simulink library "xrbsMath_r3"  (Simulink 5.0)
undefined symbols (not defined in the file or in its folder): num_width
libraries: xbsIndex_r3 x775, xrbsMath_r3 x16
(part 7 of 8)

== system xrbsMath_r3/CORDIC DIVIDER/Quadrant Map/Normalize X/Shift15 ==
  din : Inport
  cin : Inport  Port=2
  msb : Inport  Port=3
  AddSub : xbsIndex_r3/AddSub  mode=Addition  precision=Full  arith_type=Unsigned  n_bits=8  bin_pt=2  quantization=Truncate  overflow=Wrap  latency=1  explicit_period=off  period=1  en=off  dbl_ovrd=off  use_core=on  pipeline=off  use_rpm=off  gen_core=on
      settings: xl_area=[2 3 0 2 0 0 0]
  Inverter : xbsIndex_r3/Inverter  latency=0  explicit_period=off  period=1  en=off  dbl_ovrd=off
      settings: xl_area=[1 0 0 1 0 0 0]
  Inverter1 : xbsIndex_r3/Inverter  latency=0  explicit_period=off  period=1  en=off  dbl_ovrd=off
      settings: xl_area=[1 0 0 1 0 0 0]
  Logical : xbsIndex_r3/Logical  logical_function=AND  inputs=2  precision=Full  arith_type=Unsigned  n_bits=8  bin_pt=2  align_bp=on  latency=0  explicit_period=off  period=1  en=off  dbl_ovrd=off
      settings: xl_area=[1 0 0 1 0 0 0]
  Logical1 : xbsIndex_r3/Logical  logical_function=OR  inputs=2  precision=Full  arith_type=Unsigned  n_bits=8  bin_pt=2  align_bp=on  latency=0  explicit_period=off  period=1  en=off  dbl_ovrd=off
      settings: xl_area=[1 0 0 1 0 0 0]
  Mux : xbsIndex_r3/Mux  inputs=2  precision=Full  arith_type="Signed  (2's comp)"  n_bits=8  bin_pt=2  quantization=Truncate  overflow=Wrap  latency=1  mux_type=off  explicit_period=off  period=1  en=off  dbl_ovrd=off  use_rpm=off  gen_core=on
      settings: xl_area=[8 15 0 15 0 0 0]
  Register : xbsIndex_r3/Register  init=0  reg_only_valid=off  explicit_period=off  period=1  rst=off  en=off  out_en=off  dbl_ovrd=off
      settings: xl_area=[1 1 0 0 0 0 0]
  Shift : xbsIndex_r3/Shift  shift_dir=Left  shift_bits=1  precision=User Defined  arith_type=Unsigned  n_bits=num_bits  bin_pt=bin_point  quantization=Truncate  overflow=Wrap  latency=0  explicit_period=off  period=1  en=off  dbl_ovrd=off
      settings: xl_area=[0 0 0 0 0 0 0]
  Slice : xbsIndex_r3/Slice  mode=Upper Bit Location + Width  nbits=1  bit1=0  base1=MSB of Input  bit0=0  base0=LSB of Input  boolean_output=off  explicit_period=off  period=1  dbl_ovrd=off
  dout : Outport
  sum : Outport  Port=2
  latch : Outport  Port=3
  wires:
  Register/1 -> latch/1
  Shift/1 -> Mux/2
  Mux/1 -> dout/1
  Logical1/1 -> Mux/1, Register/1
  Logical/1 -> AddSub/1
  Inverter1/1 -> Logical/2
  msb/1 -> Logical1/2, Inverter1/1
  Inverter/1 -> Logical/1
  cin/1 -> AddSub/2
  AddSub/1 -> sum/1
  din/1 -> Mux/3, Shift/1, Slice/1
  Slice/1 -> Logical1/1, Inverter/1

== system xrbsMath_r3/CORDIC DIVIDER/Quadrant Map/Normalize X/Shift2 ==
  din : Inport
  cin : Inport  Port=2
  msb : Inport  Port=3
  AddSub : xbsIndex_r3/AddSub  mode=Addition  precision=Full  arith_type=Unsigned  n_bits=8  bin_pt=2  quantization=Truncate  overflow=Wrap  latency=1  explicit_period=off  period=1  en=off  dbl_ovrd=off  use_core=on  pipeline=off  use_rpm=off  gen_core=on
      settings: xl_area=[2 3 0 2 0 0 0]
  Inverter : xbsIndex_r3/Inverter  latency=0  explicit_period=off  period=1  en=off  dbl_ovrd=off
      settings: xl_area=[1 0 0 1 0 0 0]
  Inverter1 : xbsIndex_r3/Inverter  latency=0  explicit_period=off  period=1  en=off  dbl_ovrd=off
      settings: xl_area=[1 0 0 1 0 0 0]
  Logical : xbsIndex_r3/Logical  logical_function=AND  inputs=2  precision=Full  arith_type=Unsigned  n_bits=8  bin_pt=2  align_bp=on  latency=0  explicit_period=off  period=1  en=off  dbl_ovrd=off
      settings: xl_area=[1 0 0 1 0 0 0]
  Logical1 : xbsIndex_r3/Logical  logical_function=OR  inputs=2  precision=Full  arith_type=Unsigned  n_bits=8  bin_pt=2  align_bp=on  latency=0  explicit_period=off  period=1  en=off  dbl_ovrd=off
      settings: xl_area=[1 0 0 1 0 0 0]
  Mux : xbsIndex_r3/Mux  inputs=2  precision=Full  arith_type="Signed  (2's comp)"  n_bits=8  bin_pt=2  quantization=Truncate  overflow=Wrap  latency=1  mux_type=off  explicit_period=off  period=1  en=off  dbl_ovrd=off  use_rpm=off  gen_core=on
      settings: xl_area=[8 15 0 15 0 0 0]
  Register : xbsIndex_r3/Register  init=0  reg_only_valid=off  explicit_period=off  period=1  rst=off  en=off  out_en=off  dbl_ovrd=off
      settings: xl_area=[1 1 0 0 0 0 0]
  Shift : xbsIndex_r3/Shift  shift_dir=Left  shift_bits=1  precision=User Defined  arith_type=Unsigned  n_bits=num_bits  bin_pt=bin_point  quantization=Truncate  overflow=Wrap  latency=0  explicit_period=off  period=1  en=off  dbl_ovrd=off
      settings: xl_area=[0 0 0 0 0 0 0]
  Slice : xbsIndex_r3/Slice  mode=Upper Bit Location + Width  nbits=1  bit1=0  base1=MSB of Input  bit0=0  base0=LSB of Input  boolean_output=off  explicit_period=off  period=1  dbl_ovrd=off
  dout : Outport
  sum : Outport  Port=2
  latch : Outport  Port=3
  wires:
  Register/1 -> latch/1
  Shift/1 -> Mux/2
  Mux/1 -> dout/1
  Logical1/1 -> Mux/1, Register/1
  Logical/1 -> AddSub/1
  Inverter1/1 -> Logical/2
  msb/1 -> Logical1/2, Inverter1/1
  Inverter/1 -> Logical/1
  cin/1 -> AddSub/2
  AddSub/1 -> sum/1
  din/1 -> Mux/3, Shift/1, Slice/1
  Slice/1 -> Logical1/1, Inverter/1

== system xrbsMath_r3/CORDIC DIVIDER/Quadrant Map/Normalize X/Shift3 ==
  din : Inport
  cin : Inport  Port=2
  msb : Inport  Port=3
  AddSub : xbsIndex_r3/AddSub  mode=Addition  precision=Full  arith_type=Unsigned  n_bits=8  bin_pt=2  quantization=Truncate  overflow=Wrap  latency=1  explicit_period=off  period=1  en=off  dbl_ovrd=off  use_core=on  pipeline=off  use_rpm=off  gen_core=on
      settings: xl_area=[2 3 0 2 0 0 0]
  Inverter : xbsIndex_r3/Inverter  latency=0  explicit_period=off  period=1  en=off  dbl_ovrd=off
      settings: xl_area=[1 0 0 1 0 0 0]
  Inverter1 : xbsIndex_r3/Inverter  latency=0  explicit_period=off  period=1  en=off  dbl_ovrd=off
      settings: xl_area=[1 0 0 1 0 0 0]
  Logical : xbsIndex_r3/Logical  logical_function=AND  inputs=2  precision=Full  arith_type=Unsigned  n_bits=8  bin_pt=2  align_bp=on  latency=0  explicit_period=off  period=1  en=off  dbl_ovrd=off
      settings: xl_area=[1 0 0 1 0 0 0]
  Logical1 : xbsIndex_r3/Logical  logical_function=OR  inputs=2  precision=Full  arith_type=Unsigned  n_bits=8  bin_pt=2  align_bp=on  latency=0  explicit_period=off  period=1  en=off  dbl_ovrd=off
      settings: xl_area=[1 0 0 1 0 0 0]
  Mux : xbsIndex_r3/Mux  inputs=2  precision=Full  arith_type="Signed  (2's comp)"  n_bits=8  bin_pt=2  quantization=Truncate  overflow=Wrap  latency=1  mux_type=off  explicit_period=off  period=1  en=off  dbl_ovrd=off  use_rpm=off  gen_core=on
      settings: xl_area=[8 15 0 15 0 0 0]
  Register : xbsIndex_r3/Register  init=0  reg_only_valid=off  explicit_period=off  period=1  rst=off  en=off  out_en=off  dbl_ovrd=off
      settings: xl_area=[1 1 0 0 0 0 0]
  Shift : xbsIndex_r3/Shift  shift_dir=Left  shift_bits=1  precision=User Defined  arith_type=Unsigned  n_bits=num_bits  bin_pt=bin_point  quantization=Truncate  overflow=Wrap  latency=0  explicit_period=off  period=1  en=off  dbl_ovrd=off
      settings: xl_area=[0 0 0 0 0 0 0]
  Slice : xbsIndex_r3/Slice  mode=Upper Bit Location + Width  nbits=1  bit1=0  base1=MSB of Input  bit0=0  base0=LSB of Input  boolean_output=off  explicit_period=off  period=1  dbl_ovrd=off
  dout : Outport
  sum : Outport  Port=2
  latch : Outport  Port=3
  wires:
  Register/1 -> latch/1
  Shift/1 -> Mux/2
  Mux/1 -> dout/1
  Logical1/1 -> Mux/1, Register/1
  Logical/1 -> AddSub/1
  Inverter1/1 -> Logical/2
  msb/1 -> Logical1/2, Inverter1/1
  Inverter/1 -> Logical/1
  cin/1 -> AddSub/2
  AddSub/1 -> sum/1
  din/1 -> Mux/3, Shift/1, Slice/1
  Slice/1 -> Logical1/1, Inverter/1

== system xrbsMath_r3/CORDIC DIVIDER/Quadrant Map/Normalize X/Shift4 ==
  din : Inport
  cin : Inport  Port=2
  msb : Inport  Port=3
  AddSub : xbsIndex_r3/AddSub  mode=Addition  precision=Full  arith_type=Unsigned  n_bits=8  bin_pt=2  quantization=Truncate  overflow=Wrap  latency=1  explicit_period=off  period=1  en=off  dbl_ovrd=off  use_core=on  pipeline=off  use_rpm=off  gen_core=on
      settings: xl_area=[2 3 0 2 0 0 0]
  Inverter : xbsIndex_r3/Inverter  latency=0  explicit_period=off  period=1  en=off  dbl_ovrd=off
      settings: xl_area=[1 0 0 1 0 0 0]
  Inverter1 : xbsIndex_r3/Inverter  latency=0  explicit_period=off  period=1  en=off  dbl_ovrd=off
      settings: xl_area=[1 0 0 1 0 0 0]
  Logical : xbsIndex_r3/Logical  logical_function=AND  inputs=2  precision=Full  arith_type=Unsigned  n_bits=8  bin_pt=2  align_bp=on  latency=0  explicit_period=off  period=1  en=off  dbl_ovrd=off
      settings: xl_area=[1 0 0 1 0 0 0]
  Logical1 : xbsIndex_r3/Logical  logical_function=OR  inputs=2  precision=Full  arith_type=Unsigned  n_bits=8  bin_pt=2  align_bp=on  latency=0  explicit_period=off  period=1  en=off  dbl_ovrd=off
      settings: xl_area=[1 0 0 1 0 0 0]
  Mux : xbsIndex_r3/Mux  inputs=2  precision=Full  arith_type="Signed  (2's comp)"  n_bits=8  bin_pt=2  quantization=Truncate  overflow=Wrap  latency=1  mux_type=off  explicit_period=off  period=1  en=off  dbl_ovrd=off  use_rpm=off  gen_core=on
      settings: xl_area=[8 15 0 15 0 0 0]
  Register : xbsIndex_r3/Register  init=0  reg_only_valid=off  explicit_period=off  period=1  rst=off  en=off  out_en=off  dbl_ovrd=off
      settings: xl_area=[1 1 0 0 0 0 0]
  Shift : xbsIndex_r3/Shift  shift_dir=Left  shift_bits=1  precision=User Defined  arith_type=Unsigned  n_bits=num_bits  bin_pt=bin_point  quantization=Truncate  overflow=Wrap  latency=0  explicit_period=off  period=1  en=off  dbl_ovrd=off
      settings: xl_area=[0 0 0 0 0 0 0]
  Slice : xbsIndex_r3/Slice  mode=Upper Bit Location + Width  nbits=1  bit1=0  base1=MSB of Input  bit0=0  base0=LSB of Input  boolean_output=off  explicit_period=off  period=1  dbl_ovrd=off
  dout : Outport
  sum : Outport  Port=2
  latch : Outport  Port=3
  wires:
  Register/1 -> latch/1
  Shift/1 -> Mux/2
  Mux/1 -> dout/1
  Logical1/1 -> Mux/1, Register/1
  Logical/1 -> AddSub/1
  Inverter1/1 -> Logical/2
  msb/1 -> Logical1/2, Inverter1/1
  Inverter/1 -> Logical/1
  cin/1 -> AddSub/2
  AddSub/1 -> sum/1
  din/1 -> Mux/3, Shift/1, Slice/1
  Slice/1 -> Logical1/1, Inverter/1

== system xrbsMath_r3/CORDIC DIVIDER/Quadrant Map/Normalize X/Shift5 ==
  din : Inport
  cin : Inport  Port=2
  msb : Inport  Port=3
  AddSub : xbsIndex_r3/AddSub  mode=Addition  precision=Full  arith_type=Unsigned  n_bits=8  bin_pt=2  quantization=Truncate  overflow=Wrap  latency=1  explicit_period=off  period=1  en=off  dbl_ovrd=off  use_core=on  pipeline=off  use_rpm=off  gen_core=on
      settings: xl_area=[2 3 0 2 0 0 0]
  Inverter : xbsIndex_r3/Inverter  latency=0  explicit_period=off  period=1  en=off  dbl_ovrd=off
      settings: xl_area=[1 0 0 1 0 0 0]
  Inverter1 : xbsIndex_r3/Inverter  latency=0  explicit_period=off  period=1  en=off  dbl_ovrd=off
      settings: xl_area=[1 0 0 1 0 0 0]
  Logical : xbsIndex_r3/Logical  logical_function=AND  inputs=2  precision=Full  arith_type=Unsigned  n_bits=8  bin_pt=2  align_bp=on  latency=0  explicit_period=off  period=1  en=off  dbl_ovrd=off
      settings: xl_area=[1 0 0 1 0 0 0]
  Logical1 : xbsIndex_r3/Logical  logical_function=OR  inputs=2  precision=Full  arith_type=Unsigned  n_bits=8  bin_pt=2  align_bp=on  latency=0  explicit_period=off  period=1  en=off  dbl_ovrd=off
      settings: xl_area=[1 0 0 1 0 0 0]
  Mux : xbsIndex_r3/Mux  inputs=2  precision=Full  arith_type="Signed  (2's comp)"  n_bits=8  bin_pt=2  quantization=Truncate  overflow=Wrap  latency=1  mux_type=off  explicit_period=off  period=1  en=off  dbl_ovrd=off  use_rpm=off  gen_core=on
      settings: xl_area=[8 15 0 15 0 0 0]
  Register : xbsIndex_r3/Register  init=0  reg_only_valid=off  explicit_period=off  period=1  rst=off  en=off  out_en=off  dbl_ovrd=off
      settings: xl_area=[1 1 0 0 0 0 0]
  Shift : xbsIndex_r3/Shift  shift_dir=Left  shift_bits=1  precision=User Defined  arith_type=Unsigned  n_bits=num_bits  bin_pt=bin_point  quantization=Truncate  overflow=Wrap  latency=0  explicit_period=off  period=1  en=off  dbl_ovrd=off
      settings: xl_area=[0 0 0 0 0 0 0]
  Slice : xbsIndex_r3/Slice  mode=Upper Bit Location + Width  nbits=1  bit1=0  base1=MSB of Input  bit0=0  base0=LSB of Input  boolean_output=off  explicit_period=off  period=1  dbl_ovrd=off
  dout : Outport
  sum : Outport  Port=2
  latch : Outport  Port=3
  wires:
  Register/1 -> latch/1
  Shift/1 -> Mux/2
  Mux/1 -> dout/1
  Logical1/1 -> Mux/1, Register/1
  Logical/1 -> AddSub/1
  Inverter1/1 -> Logical/2
  msb/1 -> Logical1/2, Inverter1/1
  Inverter/1 -> Logical/1
  cin/1 -> AddSub/2
  AddSub/1 -> sum/1
  din/1 -> Mux/3, Shift/1, Slice/1
  Slice/1 -> Logical1/1, Inverter/1

== system xrbsMath_r3/CORDIC DIVIDER/Quadrant Map/Normalize X/Shift6 ==
  din : Inport
  cin : Inport  Port=2
  msb : Inport  Port=3
  AddSub : xbsIndex_r3/AddSub  mode=Addition  precision=Full  arith_type=Unsigned  n_bits=8  bin_pt=2  quantization=Truncate  overflow=Wrap  latency=1  explicit_period=off  period=1  en=off  dbl_ovrd=off  use_core=on  pipeline=off  use_rpm=off  gen_core=on
      settings: xl_area=[2 3 0 2 0 0 0]
  Inverter : xbsIndex_r3/Inverter  latency=0  explicit_period=off  period=1  en=off  dbl_ovrd=off
      settings: xl_area=[1 0 0 1 0 0 0]
  Inverter1 : xbsIndex_r3/Inverter  latency=0  explicit_period=off  period=1  en=off  dbl_ovrd=off
      settings: xl_area=[1 0 0 1 0 0 0]
  Logical : xbsIndex_r3/Logical  logical_function=AND  inputs=2  precision=Full  arith_type=Unsigned  n_bits=8  bin_pt=2  align_bp=on  latency=0  explicit_period=off  period=1  en=off  dbl_ovrd=off
      settings: xl_area=[1 0 0 1 0 0 0]
  Logical1 : xbsIndex_r3/Logical  logical_function=OR  inputs=2  precision=Full  arith_type=Unsigned  n_bits=8  bin_pt=2  align_bp=on  latency=0  explicit_period=off  period=1  en=off  dbl_ovrd=off
      settings: xl_area=[1 0 0 1 0 0 0]
  Mux : xbsIndex_r3/Mux  inputs=2  precision=Full  arith_type="Signed  (2's comp)"  n_bits=8  bin_pt=2  quantization=Truncate  overflow=Wrap  latency=1  mux_type=off  explicit_period=off  period=1  en=off  dbl_ovrd=off  use_rpm=off  gen_core=on
      settings: xl_area=[8 15 0 15 0 0 0]
  Register : xbsIndex_r3/Register  init=0  reg_only_valid=off  explicit_period=off  period=1  rst=off  en=off  out_en=off  dbl_ovrd=off
      settings: xl_area=[1 1 0 0 0 0 0]
  Shift : xbsIndex_r3/Shift  shift_dir=Left  shift_bits=1  precision=User Defined  arith_type=Unsigned  n_bits=num_bits  bin_pt=bin_point  quantization=Truncate  overflow=Wrap  latency=0  explicit_period=off  period=1  en=off  dbl_ovrd=off
      settings: xl_area=[0 0 0 0 0 0 0]
  Slice : xbsIndex_r3/Slice  mode=Upper Bit Location + Width  nbits=1  bit1=0  base1=MSB of Input  bit0=0  base0=LSB of Input  boolean_output=off  explicit_period=off  period=1  dbl_ovrd=off
  dout : Outport
  sum : Outport  Port=2
  latch : Outport  Port=3
  wires:
  Register/1 -> latch/1
  Shift/1 -> Mux/2
  Mux/1 -> dout/1
  Logical1/1 -> Mux/1, Register/1
  Logical/1 -> AddSub/1
  Inverter1/1 -> Logical/2
  msb/1 -> Logical1/2, Inverter1/1
  Inverter/1 -> Logical/1
  cin/1 -> AddSub/2
  AddSub/1 -> sum/1
  din/1 -> Mux/3, Shift/1, Slice/1
  Slice/1 -> Logical1/1, Inverter/1

== system xrbsMath_r3/CORDIC DIVIDER/Quadrant Map/Normalize X/Shift7 ==
  din : Inport
  cin : Inport  Port=2
  msb : Inport  Port=3
  AddSub : xbsIndex_r3/AddSub  mode=Addition  precision=Full  arith_type=Unsigned  n_bits=8  bin_pt=2  quantization=Truncate  overflow=Wrap  latency=1  explicit_period=off  period=1  en=off  dbl_ovrd=off  use_core=on  pipeline=off  use_rpm=off  gen_core=on
      settings: xl_area=[2 3 0 2 0 0 0]
  Inverter : xbsIndex_r3/Inverter  latency=0  explicit_period=off  period=1  en=off  dbl_ovrd=off
      settings: xl_area=[1 0 0 1 0 0 0]
  Inverter1 : xbsIndex_r3/Inverter  latency=0  explicit_period=off  period=1  en=off  dbl_ovrd=off
      settings: xl_area=[1 0 0 1 0 0 0]
  Logical : xbsIndex_r3/Logical  logical_function=AND  inputs=2  precision=Full  arith_type=Unsigned  n_bits=8  bin_pt=2  align_bp=on  latency=0  explicit_period=off  period=1  en=off  dbl_ovrd=off
      settings: xl_area=[1 0 0 1 0 0 0]
  Logical1 : xbsIndex_r3/Logical  logical_function=OR  inputs=2  precision=Full  arith_type=Unsigned  n_bits=8  bin_pt=2  align_bp=on  latency=0  explicit_period=off  period=1  en=off  dbl_ovrd=off
      settings: xl_area=[1 0 0 1 0 0 0]
  Mux : xbsIndex_r3/Mux  inputs=2  precision=Full  arith_type="Signed  (2's comp)"  n_bits=8  bin_pt=2  quantization=Truncate  overflow=Wrap  latency=1  mux_type=off  explicit_period=off  period=1  en=off  dbl_ovrd=off  use_rpm=off  gen_core=on
      settings: xl_area=[8 15 0 15 0 0 0]
  Register : xbsIndex_r3/Register  init=0  reg_only_valid=off  explicit_period=off  period=1  rst=off  en=off  out_en=off  dbl_ovrd=off
      settings: xl_area=[1 1 0 0 0 0 0]
  Shift : xbsIndex_r3/Shift  shift_dir=Left  shift_bits=1  precision=User Defined  arith_type=Unsigned  n_bits=num_bits  bin_pt=bin_point  quantization=Truncate  overflow=Wrap  latency=0  explicit_period=off  period=1  en=off  dbl_ovrd=off
      settings: xl_area=[0 0 0 0 0 0 0]
  Slice : xbsIndex_r3/Slice  mode=Upper Bit Location + Width  nbits=1  bit1=0  base1=MSB of Input  bit0=0  base0=LSB of Input  boolean_output=off  explicit_period=off  period=1  dbl_ovrd=off
  dout : Outport
  sum : Outport  Port=2
  latch : Outport  Port=3
  wires:
  Register/1 -> latch/1
  Shift/1 -> Mux/2
  Mux/1 -> dout/1
  Logical1/1 -> Mux/1, Register/1
  Logical/1 -> AddSub/1
  Inverter1/1 -> Logical/2
  msb/1 -> Logical1/2, Inverter1/1
  Inverter/1 -> Logical/1
  cin/1 -> AddSub/2
  AddSub/1 -> sum/1
  din/1 -> Mux/3, Shift/1, Slice/1
  Slice/1 -> Logical1/1, Inverter/1

== system xrbsMath_r3/CORDIC DIVIDER/Quadrant Map/Normalize X/Shift8 ==
  din : Inport
  cin : Inport  Port=2
  msb : Inport  Port=3
  AddSub : xbsIndex_r3/AddSub  mode=Addition  precision=Full  arith_type=Unsigned  n_bits=8  bin_pt=2  quantization=Truncate  overflow=Wrap  latency=1  explicit_period=off  period=1  en=off  dbl_ovrd=off  use_core=on  pipeline=off  use_rpm=off  gen_core=on
      settings: xl_area=[2 3 0 2 0 0 0]
  Inverter : xbsIndex_r3/Inverter  latency=0  explicit_period=off  period=1  en=off  dbl_ovrd=off
      settings: xl_area=[1 0 0 1 0 0 0]
  Inverter1 : xbsIndex_r3/Inverter  latency=0  explicit_period=off  period=1  en=off  dbl_ovrd=off
      settings: xl_area=[1 0 0 1 0 0 0]
  Logical : xbsIndex_r3/Logical  logical_function=AND  inputs=2  precision=Full  arith_type=Unsigned  n_bits=8  bin_pt=2  align_bp=on  latency=0  explicit_period=off  period=1  en=off  dbl_ovrd=off
      settings: xl_area=[1 0 0 1 0 0 0]
  Logical1 : xbsIndex_r3/Logical  logical_function=OR  inputs=2  precision=Full  arith_type=Unsigned  n_bits=8  bin_pt=2  align_bp=on  latency=0  explicit_period=off  period=1  en=off  dbl_ovrd=off
      settings: xl_area=[1 0 0 1 0 0 0]
  Mux : xbsIndex_r3/Mux  inputs=2  precision=Full  arith_type="Signed  (2's comp)"  n_bits=8  bin_pt=2  quantization=Truncate  overflow=Wrap  latency=1  mux_type=off  explicit_period=off  period=1  en=off  dbl_ovrd=off  use_rpm=off  gen_core=on
      settings: xl_area=[8 15 0 15 0 0 0]
  Register : xbsIndex_r3/Register  init=0  reg_only_valid=off  explicit_period=off  period=1  rst=off  en=off  out_en=off  dbl_ovrd=off
      settings: xl_area=[1 1 0 0 0 0 0]
  Shift : xbsIndex_r3/Shift  shift_dir=Left  shift_bits=1  precision=User Defined  arith_type=Unsigned  n_bits=num_bits  bin_pt=bin_point  quantization=Truncate  overflow=Wrap  latency=0  explicit_period=off  period=1  en=off  dbl_ovrd=off
      settings: xl_area=[0 0 0 0 0 0 0]
  Slice : xbsIndex_r3/Slice  mode=Upper Bit Location + Width  nbits=1  bit1=0  base1=MSB of Input  bit0=0  base0=LSB of Input  boolean_output=off  explicit_period=off  period=1  dbl_ovrd=off
  dout : Outport
  sum : Outport  Port=2
  latch : Outport  Port=3
  wires:
  Register/1 -> latch/1
  Shift/1 -> Mux/2
  Mux/1 -> dout/1
  Logical1/1 -> Mux/1, Register/1
  Logical/1 -> AddSub/1
  Inverter1/1 -> Logical/2
  msb/1 -> Logical1/2, Inverter1/1
  Inverter/1 -> Logical/1
  cin/1 -> AddSub/2
  AddSub/1 -> sum/1
  din/1 -> Mux/3, Shift/1, Slice/1
  Slice/1 -> Logical1/1, Inverter/1

== system xrbsMath_r3/CORDIC DIVIDER/Quadrant Map/Normalize X/Shift9 ==
  din : Inport
  cin : Inport  Port=2
  msb : Inport  Port=3
  AddSub : xbsIndex_r3/AddSub  mode=Addition  precision=Full  arith_type=Unsigned  n_bits=8  bin_pt=2  quantization=Truncate  overflow=Wrap  latency=1  explicit_period=off  period=1  en=off  dbl_ovrd=off  use_core=on  pipeline=off  use_rpm=off  gen_core=on
      settings: xl_area=[2 3 0 2 0 0 0]
  Inverter : xbsIndex_r3/Inverter  latency=0  explicit_period=off  period=1  en=off  dbl_ovrd=off
      settings: xl_area=[1 0 0 1 0 0 0]
  Inverter1 : xbsIndex_r3/Inverter  latency=0  explicit_period=off  period=1  en=off  dbl_ovrd=off
      settings: xl_area=[1 0 0 1 0 0 0]
  Logical : xbsIndex_r3/Logical  logical_function=AND  inputs=2  precision=Full  arith_type=Unsigned  n_bits=8  bin_pt=2  align_bp=on  latency=0  explicit_period=off  period=1  en=off  dbl_ovrd=off
      settings: xl_area=[1 0 0 1 0 0 0]
  Logical1 : xbsIndex_r3/Logical  logical_function=OR  inputs=2  precision=Full  arith_type=Unsigned  n_bits=8  bin_pt=2  align_bp=on  latency=0  explicit_period=off  period=1  en=off  dbl_ovrd=off
      settings: xl_area=[1 0 0 1 0 0 0]
  Mux : xbsIndex_r3/Mux  inputs=2  precision=Full  arith_type="Signed  (2's comp)"  n_bits=8  bin_pt=2  quantization=Truncate  overflow=Wrap  latency=1  mux_type=off  explicit_period=off  period=1  en=off  dbl_ovrd=off  use_rpm=off  gen_core=on
      settings: xl_area=[8 15 0 15 0 0 0]
  Register : xbsIndex_r3/Register  init=0  reg_only_valid=off  explicit_period=off  period=1  rst=off  en=off  out_en=off  dbl_ovrd=off
      settings: xl_area=[1 1 0 0 0 0 0]
  Shift : xbsIndex_r3/Shift  shift_dir=Left  shift_bits=1  precision=User Defined  arith_type=Unsigned  n_bits=num_bits  bin_pt=bin_point  quantization=Truncate  overflow=Wrap  latency=0  explicit_period=off  period=1  en=off  dbl_ovrd=off
      settings: xl_area=[0 0 0 0 0 0 0]
  Slice : xbsIndex_r3/Slice  mode=Upper Bit Location + Width  nbits=1  bit1=0  base1=MSB of Input  bit0=0  base0=LSB of Input  boolean_output=off  explicit_period=off  period=1  dbl_ovrd=off
  dout : Outport
  sum : Outport  Port=2
  latch : Outport  Port=3
  wires:
  Register/1 -> latch/1
  Shift/1 -> Mux/2
  Mux/1 -> dout/1
  Logical1/1 -> Mux/1, Register/1
  Logical/1 -> AddSub/1
  Inverter1/1 -> Logical/2
  msb/1 -> Logical1/2, Inverter1/1
  Inverter/1 -> Logical/1
  cin/1 -> AddSub/2
  AddSub/1 -> sum/1
  din/1 -> Mux/3, Shift/1, Slice/1
  Slice/1 -> Logical1/1, Inverter/1

== system xrbsMath_r3/CORDIC DIVIDER/Quadrant Map/Normalize Y/Shift1 ==
  din : Inport
  cin : Inport  Port=2
  msb : Inport  Port=3
  AddSub : xbsIndex_r3/AddSub  mode=Addition  precision=Full  arith_type=Unsigned  n_bits=8  bin_pt=2  quantization=Truncate  overflow=Wrap  latency=1  explicit_period=off  period=1  en=off  dbl_ovrd=off  use_core=on  pipeline=off  use_rpm=off  gen_core=on
      settings: xl_area=[2 3 0 2 0 0 0]
  Inverter : xbsIndex_r3/Inverter  latency=0  explicit_period=off  period=1  en=off  dbl_ovrd=off
      settings: xl_area=[1 0 0 1 0 0 0]
  Inverter1 : xbsIndex_r3/Inverter  latency=0  explicit_period=off  period=1  en=off  dbl_ovrd=off
      settings: xl_area=[1 0 0 1 0 0 0]
  Logical : xbsIndex_r3/Logical  logical_function=AND  inputs=2  precision=Full  arith_type=Unsigned  n_bits=8  bin_pt=2  align_bp=on  latency=0  explicit_period=off  period=1  en=off  dbl_ovrd=off
      settings: xl_area=[1 0 0 1 0 0 0]
  Logical1 : xbsIndex_r3/Logical  logical_function=OR  inputs=2  precision=Full  arith_type=Unsigned  n_bits=8  bin_pt=2  align_bp=on  latency=0  explicit_period=off  period=1  en=off  dbl_ovrd=off
      settings: xl_area=[1 0 0 1 0 0 0]
  Mux : xbsIndex_r3/Mux  inputs=2  precision=Full  arith_type="Signed  (2's comp)"  n_bits=8  bin_pt=2  quantization=Truncate  overflow=Wrap  latency=1  mux_type=off  explicit_period=off  period=1  en=off  dbl_ovrd=off  use_rpm=off  gen_core=on
      settings: xl_area=[8 15 0 15 0 0 0]
  Register : xbsIndex_r3/Register  init=0  reg_only_valid=off  explicit_period=off  period=1  rst=off  en=off  out_en=off  dbl_ovrd=off
      settings: xl_area=[1 1 0 0 0 0 0]
  Shift : xbsIndex_r3/Shift  shift_dir=Left  shift_bits=1  precision=User Defined  arith_type=Unsigned  n_bits=num_bits  bin_pt=bin_point  quantization=Truncate  overflow=Wrap  latency=0  explicit_period=off  period=1  en=off  dbl_ovrd=off
      settings: xl_area=[0 0 0 0 0 0 0]
  Slice : xbsIndex_r3/Slice  mode=Upper Bit Location + Width  nbits=1  bit1=0  base1=MSB of Input  bit0=0  base0=LSB of Input  boolean_output=off  explicit_period=off  period=1  dbl_ovrd=off
  dout : Outport
  sum : Outport  Port=2
  latch : Outport  Port=3
  wires:
  Register/1 -> latch/1
  Shift/1 -> Mux/2
  Mux/1 -> dout/1
  Logical1/1 -> Mux/1, Register/1
  Logical/1 -> AddSub/1
  Inverter1/1 -> Logical/2
  msb/1 -> Logical1/2, Inverter1/1
  Inverter/1 -> Logical/1
  cin/1 -> AddSub/2
  AddSub/1 -> sum/1
  din/1 -> Mux/3, Shift/1, Slice/1
  Slice/1 -> Logical1/1, Inverter/1

== system xrbsMath_r3/CORDIC DIVIDER/Quadrant Map/Normalize Y/Shift10 ==
  din : Inport
  cin : Inport  Port=2
  msb : Inport  Port=3
  AddSub : xbsIndex_r3/AddSub  mode=Addition  precision=Full  arith_type=Unsigned  n_bits=8  bin_pt=2  quantization=Truncate  overflow=Wrap  latency=1  explicit_period=off  period=1  en=off  dbl_ovrd=off  use_core=on  pipeline=off  use_rpm=off  gen_core=on
      settings: xl_area=[2 3 0 2 0 0 0]
  Inverter : xbsIndex_r3/Inverter  latency=0  explicit_period=off  period=1  en=off  dbl_ovrd=off
      settings: xl_area=[1 0 0 1 0 0 0]
  Inverter1 : xbsIndex_r3/Inverter  latency=0  explicit_period=off  period=1  en=off  dbl_ovrd=off
      settings: xl_area=[1 0 0 1 0 0 0]
  Logical : xbsIndex_r3/Logical  logical_function=AND  inputs=2  precision=Full  arith_type=Unsigned  n_bits=8  bin_pt=2  align_bp=on  latency=0  explicit_period=off  period=1  en=off  dbl_ovrd=off
      settings: xl_area=[1 0 0 1 0 0 0]
  Logical1 : xbsIndex_r3/Logical  logical_function=OR  inputs=2  precision=Full  arith_type=Unsigned  n_bits=8  bin_pt=2  align_bp=on  latency=0  explicit_period=off  period=1  en=off  dbl_ovrd=off
      settings: xl_area=[1 0 0 1 0 0 0]
  Mux : xbsIndex_r3/Mux  inputs=2  precision=Full  arith_type="Signed  (2's comp)"  n_bits=8  bin_pt=2  quantization=Truncate  overflow=Wrap  latency=1  mux_type=off  explicit_period=off  period=1  en=off  dbl_ovrd=off  use_rpm=off  gen_core=on
      settings: xl_area=[8 15 0 15 0 0 0]
  Register : xbsIndex_r3/Register  init=0  reg_only_valid=off  explicit_period=off  period=1  rst=off  en=off  out_en=off  dbl_ovrd=off
      settings: xl_area=[1 1 0 0 0 0 0]
  Shift : xbsIndex_r3/Shift  shift_dir=Left  shift_bits=1  precision=User Defined  arith_type=Unsigned  n_bits=num_bits  bin_pt=bin_point  quantization=Truncate  overflow=Wrap  latency=0  explicit_period=off  period=1  en=off  dbl_ovrd=off
      settings: xl_area=[0 0 0 0 0 0 0]
  Slice : xbsIndex_r3/Slice  mode=Upper Bit Location + Width  nbits=1  bit1=0  base1=MSB of Input  bit0=0  base0=LSB of Input  boolean_output=off  explicit_period=off  period=1  dbl_ovrd=off
  dout : Outport
  sum : Outport  Port=2
  latch : Outport  Port=3
  wires:
  Slice/1 -> Inverter/1, Logical1/1
  din/1 -> Slice/1, Shift/1, Mux/3
  AddSub/1 -> sum/1
  cin/1 -> AddSub/2
  Inverter/1 -> Logical/1
  msb/1 -> Inverter1/1, Logical1/2
  Inverter1/1 -> Logical/2
  Logical/1 -> AddSub/1
  Logical1/1 -> Register/1, Mux/1
  Mux/1 -> dout/1
  Shift/1 -> Mux/2
  Register/1 -> latch/1

== system xrbsMath_r3/CORDIC DIVIDER/Quadrant Map/Normalize Y/Shift11 ==
  din : Inport
  cin : Inport  Port=2
  msb : Inport  Port=3
  AddSub : xbsIndex_r3/AddSub  mode=Addition  precision=Full  arith_type=Unsigned  n_bits=8  bin_pt=2  quantization=Truncate  overflow=Wrap  latency=1  explicit_period=off  period=1  en=off  dbl_ovrd=off  use_core=on  pipeline=off  use_rpm=off  gen_core=on
      settings: xl_area=[2 3 0 2 0 0 0]
  Inverter : xbsIndex_r3/Inverter  latency=0  explicit_period=off  period=1  en=off  dbl_ovrd=off
      settings: xl_area=[1 0 0 1 0 0 0]
  Inverter1 : xbsIndex_r3/Inverter  latency=0  explicit_period=off  period=1  en=off  dbl_ovrd=off
      settings: xl_area=[1 0 0 1 0 0 0]
  Logical : xbsIndex_r3/Logical  logical_function=AND  inputs=2  precision=Full  arith_type=Unsigned  n_bits=8  bin_pt=2  align_bp=on  latency=0  explicit_period=off  period=1  en=off  dbl_ovrd=off
      settings: xl_area=[1 0 0 1 0 0 0]
  Logical1 : xbsIndex_r3/Logical  logical_function=OR  inputs=2  precision=Full  arith_type=Unsigned  n_bits=8  bin_pt=2  align_bp=on  latency=0  explicit_period=off  period=1  en=off  dbl_ovrd=off
      settings: xl_area=[1 0 0 1 0 0 0]
  Mux : xbsIndex_r3/Mux  inputs=2  precision=Full  arith_type="Signed  (2's comp)"  n_bits=8  bin_pt=2  quantization=Truncate  overflow=Wrap  latency=1  mux_type=off  explicit_period=off  period=1  en=off  dbl_ovrd=off  use_rpm=off  gen_core=on
      settings: xl_area=[8 15 0 15 0 0 0]
  Register : xbsIndex_r3/Register  init=0  reg_only_valid=off  explicit_period=off  period=1  rst=off  en=off  out_en=off  dbl_ovrd=off
      settings: xl_area=[1 1 0 0 0 0 0]
  Shift : xbsIndex_r3/Shift  shift_dir=Left  shift_bits=1  precision=User Defined  arith_type=Unsigned  n_bits=num_bits  bin_pt=bin_point  quantization=Truncate  overflow=Wrap  latency=0  explicit_period=off  period=1  en=off  dbl_ovrd=off
      settings: xl_area=[0 0 0 0 0 0 0]
  Slice : xbsIndex_r3/Slice  mode=Upper Bit Location + Width  nbits=1  bit1=0  base1=MSB of Input  bit0=0  base0=LSB of Input  boolean_output=off  explicit_period=off  period=1  dbl_ovrd=off
  dout : Outport
  sum : Outport  Port=2
  latch : Outport  Port=3
  wires:
  Slice/1 -> Inverter/1, Logical1/1
  din/1 -> Slice/1, Shift/1, Mux/3
  AddSub/1 -> sum/1
  cin/1 -> AddSub/2
  Inverter/1 -> Logical/1
  msb/1 -> Inverter1/1, Logical1/2
  Inverter1/1 -> Logical/2
  Logical/1 -> AddSub/1
  Logical1/1 -> Register/1, Mux/1
  Mux/1 -> dout/1
  Shift/1 -> Mux/2
  Register/1 -> latch/1

== system xrbsMath_r3/CORDIC DIVIDER/Quadrant Map/Normalize Y/Shift12 ==
  din : Inport
  cin : Inport  Port=2
  msb : Inport  Port=3
  AddSub : xbsIndex_r3/AddSub  mode=Addition  precision=Full  arith_type=Unsigned  n_bits=8  bin_pt=2  quantization=Truncate  overflow=Wrap  latency=1  explicit_period=off  period=1  en=off  dbl_ovrd=off  use_core=on  pipeline=off  use_rpm=off  gen_core=on
      settings: xl_area=[2 3 0 2 0 0 0]
  Inverter : xbsIndex_r3/Inverter  latency=0  explicit_period=off  period=1  en=off  dbl_ovrd=off
      settings: xl_area=[1 0 0 1 0 0 0]
  Inverter1 : xbsIndex_r3/Inverter  latency=0  explicit_period=off  period=1  en=off  dbl_ovrd=off
      settings: xl_area=[1 0 0 1 0 0 0]
  Logical : xbsIndex_r3/Logical  logical_function=AND  inputs=2  precision=Full  arith_type=Unsigned  n_bits=8  bin_pt=2  align_bp=on  latency=0  explicit_period=off  period=1  en=off  dbl_ovrd=off
      settings: xl_area=[1 0 0 1 0 0 0]
  Logical1 : xbsIndex_r3/Logical  logical_function=OR  inputs=2  precision=Full  arith_type=Unsigned  n_bits=8  bin_pt=2  align_bp=on  latency=0  explicit_period=off  period=1  en=off  dbl_ovrd=off
      settings: xl_area=[1 0 0 1 0 0 0]
  Mux : xbsIndex_r3/Mux  inputs=2  precision=Full  arith_type="Signed  (2's comp)"  n_bits=8  bin_pt=2  quantization=Truncate  overflow=Wrap  latency=1  mux_type=off  explicit_period=off  period=1  en=off  dbl_ovrd=off  use_rpm=off  gen_core=on
      settings: xl_area=[8 15 0 15 0 0 0]
  Register : xbsIndex_r3/Register  init=0  reg_only_valid=off  explicit_period=off  period=1  rst=off  en=off  out_en=off  dbl_ovrd=off
      settings: xl_area=[1 1 0 0 0 0 0]
  Shift : xbsIndex_r3/Shift  shift_dir=Left  shift_bits=1  precision=User Defined  arith_type=Unsigned  n_bits=num_bits  bin_pt=bin_point  quantization=Truncate  overflow=Wrap  latency=0  explicit_period=off  period=1  en=off  dbl_ovrd=off
      settings: xl_area=[0 0 0 0 0 0 0]
  Slice : xbsIndex_r3/Slice  mode=Upper Bit Location + Width  nbits=1  bit1=0  base1=MSB of Input  bit0=0  base0=LSB of Input  boolean_output=off  explicit_period=off  period=1  dbl_ovrd=off
  dout : Outport
  sum : Outport  Port=2
  latch : Outport  Port=3
  wires:
  Slice/1 -> Inverter/1, Logical1/1
  din/1 -> Slice/1, Shift/1, Mux/3
  AddSub/1 -> sum/1
  cin/1 -> AddSub/2
  Inverter/1 -> Logical/1
  msb/1 -> Inverter1/1, Logical1/2
  Inverter1/1 -> Logical/2
  Logical/1 -> AddSub/1
  Logical1/1 -> Register/1, Mux/1
  Mux/1 -> dout/1
  Shift/1 -> Mux/2
  Register/1 -> latch/1

== system xrbsMath_r3/CORDIC DIVIDER/Quadrant Map/Normalize Y/Shift13 ==
  din : Inport
  cin : Inport  Port=2
  msb : Inport  Port=3
  AddSub : xbsIndex_r3/AddSub  mode=Addition  precision=Full  arith_type=Unsigned  n_bits=8  bin_pt=2  quantization=Truncate  overflow=Wrap  latency=1  explicit_period=off  period=1  en=off  dbl_ovrd=off  use_core=on  pipeline=off  use_rpm=off  gen_core=on
      settings: xl_area=[2 3 0 2 0 0 0]
  Inverter : xbsIndex_r3/Inverter  latency=0  explicit_period=off  period=1  en=off  dbl_ovrd=off
      settings: xl_area=[1 0 0 1 0 0 0]
  Inverter1 : xbsIndex_r3/Inverter  latency=0  explicit_period=off  period=1  en=off  dbl_ovrd=off
      settings: xl_area=[1 0 0 1 0 0 0]
  Logical : xbsIndex_r3/Logical  logical_function=AND  inputs=2  precision=Full  arith_type=Unsigned  n_bits=8  bin_pt=2  align_bp=on  latency=0  explicit_period=off  period=1  en=off  dbl_ovrd=off
      settings: xl_area=[1 0 0 1 0 0 0]
  Logical1 : xbsIndex_r3/Logical  logical_function=OR  inputs=2  precision=Full  arith_type=Unsigned  n_bits=8  bin_pt=2  align_bp=on  latency=0  explicit_period=off  period=1  en=off  dbl_ovrd=off
      settings: xl_area=[1 0 0 1 0 0 0]
  Mux : xbsIndex_r3/Mux  inputs=2  precision=Full  arith_type="Signed  (2's comp)"  n_bits=8  bin_pt=2  quantization=Truncate  overflow=Wrap  latency=1  mux_type=off  explicit_period=off  period=1  en=off  dbl_ovrd=off  use_rpm=off  gen_core=on
      settings: xl_area=[8 15 0 15 0 0 0]
  Register : xbsIndex_r3/Register  init=0  reg_only_valid=off  explicit_period=off  period=1  rst=off  en=off  out_en=off  dbl_ovrd=off
      settings: xl_area=[1 1 0 0 0 0 0]
  Shift : xbsIndex_r3/Shift  shift_dir=Left  shift_bits=1  precision=User Defined  arith_type=Unsigned  n_bits=num_bits  bin_pt=bin_point  quantization=Truncate  overflow=Wrap  latency=0  explicit_period=off  period=1  en=off  dbl_ovrd=off
      settings: xl_area=[0 0 0 0 0 0 0]
  Slice : xbsIndex_r3/Slice  mode=Upper Bit Location + Width  nbits=1  bit1=0  base1=MSB of Input  bit0=0  base0=LSB of Input  boolean_output=off  explicit_period=off  period=1  dbl_ovrd=off
  dout : Outport
  sum : Outport  Port=2
  latch : Outport  Port=3
  wires:
  Slice/1 -> Inverter/1, Logical1/1
  din/1 -> Slice/1, Shift/1, Mux/3
  AddSub/1 -> sum/1
  cin/1 -> AddSub/2
  Inverter/1 -> Logical/1
  msb/1 -> Inverter1/1, Logical1/2
  Inverter1/1 -> Logical/2
  Logical/1 -> AddSub/1
  Logical1/1 -> Register/1, Mux/1
  Mux/1 -> dout/1
  Shift/1 -> Mux/2
  Register/1 -> latch/1

== system xrbsMath_r3/CORDIC DIVIDER/Quadrant Map/Normalize Y/Shift14 ==
  din : Inport
  cin : Inport  Port=2
  msb : Inport  Port=3
  AddSub : xbsIndex_r3/AddSub  mode=Addition  precision=Full  arith_type=Unsigned  n_bits=8  bin_pt=2  quantization=Truncate  overflow=Wrap  latency=1  explicit_period=off  period=1  en=off  dbl_ovrd=off  use_core=on  pipeline=off  use_rpm=off  gen_core=on
      settings: xl_area=[2 3 0 2 0 0 0]
  Inverter : xbsIndex_r3/Inverter  latency=0  explicit_period=off  period=1  en=off  dbl_ovrd=off
      settings: xl_area=[1 0 0 1 0 0 0]
  Inverter1 : xbsIndex_r3/Inverter  latency=0  explicit_period=off  period=1  en=off  dbl_ovrd=off
      settings: xl_area=[1 0 0 1 0 0 0]
  Logical : xbsIndex_r3/Logical  logical_function=AND  inputs=2  precision=Full  arith_type=Unsigned  n_bits=8  bin_pt=2  align_bp=on  latency=0  explicit_period=off  period=1  en=off  dbl_ovrd=off
      settings: xl_area=[1 0 0 1 0 0 0]
  Logical1 : xbsIndex_r3/Logical  logical_function=OR  inputs=2  precision=Full  arith_type=Unsigned  n_bits=8  bin_pt=2  align_bp=on  latency=0  explicit_period=off  period=1  en=off  dbl_ovrd=off
      settings: xl_area=[1 0 0 1 0 0 0]
  Mux : xbsIndex_r3/Mux  inputs=2  precision=Full  arith_type="Signed  (2's comp)"  n_bits=8  bin_pt=2  quantization=Truncate  overflow=Wrap  latency=1  mux_type=off  explicit_period=off  period=1  en=off  dbl_ovrd=off  use_rpm=off  gen_core=on
      settings: xl_area=[8 15 0 15 0 0 0]
  Register : xbsIndex_r3/Register  init=0  reg_only_valid=off  explicit_period=off  period=1  rst=off  en=off  out_en=off  dbl_ovrd=off
      settings: xl_area=[1 1 0 0 0 0 0]
  Shift : xbsIndex_r3/Shift  shift_dir=Left  shift_bits=1  precision=User Defined  arith_type=Unsigned  n_bits=num_bits  bin_pt=bin_point  quantization=Truncate  overflow=Wrap  latency=0  explicit_period=off  period=1  en=off  dbl_ovrd=off
      settings: xl_area=[0 0 0 0 0 0 0]
  Slice : xbsIndex_r3/Slice  mode=Upper Bit Location + Width  nbits=1  bit1=0  base1=MSB of Input  bit0=0  base0=LSB of Input  boolean_output=off  explicit_period=off  period=1  dbl_ovrd=off
  dout : Outport
  sum : Outport  Port=2
  latch : Outport  Port=3
  wires:
  Slice/1 -> Inverter/1, Logical1/1
  din/1 -> Slice/1, Shift/1, Mux/3
  AddSub/1 -> sum/1
  cin/1 -> AddSub/2
  Inverter/1 -> Logical/1
  msb/1 -> Inverter1/1, Logical1/2
  Inverter1/1 -> Logical/2
  Logical/1 -> AddSub/1
  Logical1/1 -> Register/1, Mux/1
  Mux/1 -> dout/1
  Shift/1 -> Mux/2
  Register/1 -> latch/1

== system xrbsMath_r3/CORDIC DIVIDER/Quadrant Map/Normalize Y/Shift15 ==
  din : Inport
  cin : Inport  Port=2
  msb : Inport  Port=3
  AddSub : xbsIndex_r3/AddSub  mode=Addition  precision=Full  arith_type=Unsigned  n_bits=8  bin_pt=2  quantization=Truncate  overflow=Wrap  latency=1  explicit_period=off  period=1  en=off  dbl_ovrd=off  use_core=on  pipeline=off  use_rpm=off  gen_core=on
      settings: xl_area=[2 3 0 2 0 0 0]
  Inverter : xbsIndex_r3/Inverter  latency=0  explicit_period=off  period=1  en=off  dbl_ovrd=off
      settings: xl_area=[1 0 0 1 0 0 0]
  Inverter1 : xbsIndex_r3/Inverter  latency=0  explicit_period=off  period=1  en=off  dbl_ovrd=off
      settings: xl_area=[1 0 0 1 0 0 0]
  Logical : xbsIndex_r3/Logical  logical_function=AND  inputs=2  precision=Full  arith_type=Unsigned  n_bits=8  bin_pt=2  align_bp=on  latency=0  explicit_period=off  period=1  en=off  dbl_ovrd=off
      settings: xl_area=[1 0 0 1 0 0 0]
  Logical1 : xbsIndex_r3/Logical  logical_function=OR  inputs=2  precision=Full  arith_type=Unsigned  n_bits=8  bin_pt=2  align_bp=on  latency=0  explicit_period=off  period=1  en=off  dbl_ovrd=off
      settings: xl_area=[1 0 0 1 0 0 0]
  Mux : xbsIndex_r3/Mux  inputs=2  precision=Full  arith_type="Signed  (2's comp)"  n_bits=8  bin_pt=2  quantization=Truncate  overflow=Wrap  latency=1  mux_type=off  explicit_period=off  period=1  en=off  dbl_ovrd=off  use_rpm=off  gen_core=on
      settings: xl_area=[8 15 0 15 0 0 0]
  Register : xbsIndex_r3/Register  init=0  reg_only_valid=off  explicit_period=off  period=1  rst=off  en=off  out_en=off  dbl_ovrd=off
      settings: xl_area=[1 1 0 0 0 0 0]
  Shift : xbsIndex_r3/Shift  shift_dir=Left  shift_bits=1  precision=User Defined  arith_type=Unsigned  n_bits=num_bits  bin_pt=bin_point  quantization=Truncate  overflow=Wrap  latency=0  explicit_period=off  period=1  en=off  dbl_ovrd=off
      settings: xl_area=[0 0 0 0 0 0 0]
  Slice : xbsIndex_r3/Slice  mode=Upper Bit Location + Width  nbits=1  bit1=0  base1=MSB of Input  bit0=0  base0=LSB of Input  boolean_output=off  explicit_period=off  period=1  dbl_ovrd=off
  dout : Outport
  sum : Outport  Port=2
  latch : Outport  Port=3
  wires:
  Slice/1 -> Inverter/1, Logical1/1
  din/1 -> Slice/1, Shift/1, Mux/3
  AddSub/1 -> sum/1
  cin/1 -> AddSub/2
  Inverter/1 -> Logical/1
  msb/1 -> Inverter1/1, Logical1/2
  Inverter1/1 -> Logical/2
  Logical/1 -> AddSub/1
  Logical1/1 -> Register/1, Mux/1
  Mux/1 -> dout/1
  Shift/1 -> Mux/2
  Register/1 -> latch/1

== system xrbsMath_r3/CORDIC DIVIDER/Quadrant Map/Normalize Y/Shift2 ==
  din : Inport
  cin : Inport  Port=2
  msb : Inport  Port=3
  AddSub : xbsIndex_r3/AddSub  mode=Addition  precision=Full  arith_type=Unsigned  n_bits=8  bin_pt=2  quantization=Truncate  overflow=Wrap  latency=1  explicit_period=off  period=1  en=off  dbl_ovrd=off  use_core=on  pipeline=off  use_rpm=off  gen_core=on
      settings: xl_area=[2 3 0 2 0 0 0]
  Inverter : xbsIndex_r3/Inverter  latency=0  explicit_period=off  period=1  en=off  dbl_ovrd=off
      settings: xl_area=[1 0 0 1 0 0 0]
  Inverter1 : xbsIndex_r3/Inverter  latency=0  explicit_period=off  period=1  en=off  dbl_ovrd=off
      settings: xl_area=[1 0 0 1 0 0 0]
  Logical : xbsIndex_r3/Logical  logical_function=AND  inputs=2  precision=Full  arith_type=Unsigned  n_bits=8  bin_pt=2  align_bp=on  latency=0  explicit_period=off  period=1  en=off  dbl_ovrd=off
      settings: xl_area=[1 0 0 1 0 0 0]
  Logical1 : xbsIndex_r3/Logical  logical_function=OR  inputs=2  precision=Full  arith_type=Unsigned  n_bits=8  bin_pt=2  align_bp=on  latency=0  explicit_period=off  period=1  en=off  dbl_ovrd=off
      settings: xl_area=[1 0 0 1 0 0 0]
  Mux : xbsIndex_r3/Mux  inputs=2  precision=Full  arith_type="Signed  (2's comp)"  n_bits=8  bin_pt=2  quantization=Truncate  overflow=Wrap  latency=1  mux_type=off  explicit_period=off  period=1  en=off  dbl_ovrd=off  use_rpm=off  gen_core=on
      settings: xl_area=[8 15 0 15 0 0 0]
  Register : xbsIndex_r3/Register  init=0  reg_only_valid=off  explicit_period=off  period=1  rst=off  en=off  out_en=off  dbl_ovrd=off
      settings: xl_area=[1 1 0 0 0 0 0]
  Shift : xbsIndex_r3/Shift  shift_dir=Left  shift_bits=1  precision=User Defined  arith_type=Unsigned  n_bits=num_bits  bin_pt=bin_point  quantization=Truncate  overflow=Wrap  latency=0  explicit_period=off  period=1  en=off  dbl_ovrd=off
      settings: xl_area=[0 0 0 0 0 0 0]
  Slice : xbsIndex_r3/Slice  mode=Upper Bit Location + Width  nbits=1  bit1=0  base1=MSB of Input  bit0=0  base0=LSB of Input  boolean_output=off  explicit_period=off  period=1  dbl_ovrd=off
  dout : Outport
  sum : Outport  Port=2
  latch : Outport  Port=3
  wires:
  Slice/1 -> Inverter/1, Logical1/1
  din/1 -> Slice/1, Shift/1, Mux/3
  AddSub/1 -> sum/1
  cin/1 -> AddSub/2
  Inverter/1 -> Logical/1
  msb/1 -> Inverter1/1, Logical1/2
  Inverter1/1 -> Logical/2
  Logical/1 -> AddSub/1
  Logical1/1 -> Register/1, Mux/1
  Mux/1 -> dout/1
  Shift/1 -> Mux/2
  Register/1 -> latch/1

== system xrbsMath_r3/CORDIC DIVIDER/Quadrant Map/Normalize Y/Shift3 ==
  din : Inport
  cin : Inport  Port=2
  msb : Inport  Port=3
  AddSub : xbsIndex_r3/AddSub  mode=Addition  precision=Full  arith_type=Unsigned  n_bits=8  bin_pt=2  quantization=Truncate  overflow=Wrap  latency=1  explicit_period=off  period=1  en=off  dbl_ovrd=off  use_core=on  pipeline=off  use_rpm=off  gen_core=on
      settings: xl_area=[2 3 0 2 0 0 0]
  Inverter : xbsIndex_r3/Inverter  latency=0  explicit_period=off  period=1  en=off  dbl_ovrd=off
      settings: xl_area=[1 0 0 1 0 0 0]
  Inverter1 : xbsIndex_r3/Inverter  latency=0  explicit_period=off  period=1  en=off  dbl_ovrd=off
      settings: xl_area=[1 0 0 1 0 0 0]
  Logical : xbsIndex_r3/Logical  logical_function=AND  inputs=2  precision=Full  arith_type=Unsigned  n_bits=8  bin_pt=2  align_bp=on  latency=0  explicit_period=off  period=1  en=off  dbl_ovrd=off
      settings: xl_area=[1 0 0 1 0 0 0]
  Logical1 : xbsIndex_r3/Logical  logical_function=OR  inputs=2  precision=Full  arith_type=Unsigned  n_bits=8  bin_pt=2  align_bp=on  latency=0  explicit_period=off  period=1  en=off  dbl_ovrd=off
      settings: xl_area=[1 0 0 1 0 0 0]
  Mux : xbsIndex_r3/Mux  inputs=2  precision=Full  arith_type="Signed  (2's comp)"  n_bits=8  bin_pt=2  quantization=Truncate  overflow=Wrap  latency=1  mux_type=off  explicit_period=off  period=1  en=off  dbl_ovrd=off  use_rpm=off  gen_core=on
      settings: xl_area=[8 15 0 15 0 0 0]
  Register : xbsIndex_r3/Register  init=0  reg_only_valid=off  explicit_period=off  period=1  rst=off  en=off  out_en=off  dbl_ovrd=off
      settings: xl_area=[1 1 0 0 0 0 0]
  Shift : xbsIndex_r3/Shift  shift_dir=Left  shift_bits=1  precision=User Defined  arith_type=Unsigned  n_bits=num_bits  bin_pt=bin_point  quantization=Truncate  overflow=Wrap  latency=0  explicit_period=off  period=1  en=off  dbl_ovrd=off
      settings: xl_area=[0 0 0 0 0 0 0]
  Slice : xbsIndex_r3/Slice  mode=Upper Bit Location + Width  nbits=1  bit1=0  base1=MSB of Input  bit0=0  base0=LSB of Input  boolean_output=off  explicit_period=off  period=1  dbl_ovrd=off
  dout : Outport
  sum : Outport  Port=2
  latch : Outport  Port=3
  wires:
  Slice/1 -> Inverter/1, Logical1/1
  din/1 -> Slice/1, Shift/1, Mux/3
  AddSub/1 -> sum/1
  cin/1 -> AddSub/2
  Inverter/1 -> Logical/1
  msb/1 -> Inverter1/1, Logical1/2
  Inverter1/1 -> Logical/2
  Logical/1 -> AddSub/1
  Logical1/1 -> Register/1, Mux/1
  Mux/1 -> dout/1
  Shift/1 -> Mux/2
  Register/1 -> latch/1

== system xrbsMath_r3/CORDIC DIVIDER/Quadrant Map/Normalize Y/Shift4 ==
  din : Inport
  cin : Inport  Port=2
  msb : Inport  Port=3
  AddSub : xbsIndex_r3/AddSub  mode=Addition  precision=Full  arith_type=Unsigned  n_bits=8  bin_pt=2  quantization=Truncate  overflow=Wrap  latency=1  explicit_period=off  period=1  en=off  dbl_ovrd=off  use_core=on  pipeline=off  use_rpm=off  gen_core=on
      settings: xl_area=[2 3 0 2 0 0 0]
  Inverter : xbsIndex_r3/Inverter  latency=0  explicit_period=off  period=1  en=off  dbl_ovrd=off
      settings: xl_area=[1 0 0 1 0 0 0]
  Inverter1 : xbsIndex_r3/Inverter  latency=0  explicit_period=off  period=1  en=off  dbl_ovrd=off
      settings: xl_area=[1 0 0 1 0 0 0]
  Logical : xbsIndex_r3/Logical  logical_function=AND  inputs=2  precision=Full  arith_type=Unsigned  n_bits=8  bin_pt=2  align_bp=on  latency=0  explicit_period=off  period=1  en=off  dbl_ovrd=off
      settings: xl_area=[1 0 0 1 0 0 0]
  Logical1 : xbsIndex_r3/Logical  logical_function=OR  inputs=2  precision=Full  arith_type=Unsigned  n_bits=8  bin_pt=2  align_bp=on  latency=0  explicit_period=off  period=1  en=off  dbl_ovrd=off
      settings: xl_area=[1 0 0 1 0 0 0]
  Mux : xbsIndex_r3/Mux  inputs=2  precision=Full  arith_type="Signed  (2's comp)"  n_bits=8  bin_pt=2  quantization=Truncate  overflow=Wrap  latency=1  mux_type=off  explicit_period=off  period=1  en=off  dbl_ovrd=off  use_rpm=off  gen_core=on
      settings: xl_area=[8 15 0 15 0 0 0]
  Register : xbsIndex_r3/Register  init=0  reg_only_valid=off  explicit_period=off  period=1  rst=off  en=off  out_en=off  dbl_ovrd=off
      settings: xl_area=[1 1 0 0 0 0 0]
  Shift : xbsIndex_r3/Shift  shift_dir=Left  shift_bits=1  precision=User Defined  arith_type=Unsigned  n_bits=num_bits  bin_pt=bin_point  quantization=Truncate  overflow=Wrap  latency=0  explicit_period=off  period=1  en=off  dbl_ovrd=off
      settings: xl_area=[0 0 0 0 0 0 0]
  Slice : xbsIndex_r3/Slice  mode=Upper Bit Location + Width  nbits=1  bit1=0  base1=MSB of Input  bit0=0  base0=LSB of Input  boolean_output=off  explicit_period=off  period=1  dbl_ovrd=off
  dout : Outport
  sum : Outport  Port=2
  latch : Outport  Port=3
  wires:
  Slice/1 -> Inverter/1, Logical1/1
  din/1 -> Slice/1, Shift/1, Mux/3
  AddSub/1 -> sum/1
  cin/1 -> AddSub/2
  Inverter/1 -> Logical/1
  msb/1 -> Inverter1/1, Logical1/2
  Inverter1/1 -> Logical/2
  Logical/1 -> AddSub/1
  Logical1/1 -> Register/1, Mux/1
  Mux/1 -> dout/1
  Shift/1 -> Mux/2
  Register/1 -> latch/1
